simulink library "halout"  (R2021b)
settings: Solver=VariableStepAuto  StartTime=0.0  StopTime=10.0  RelTol=1e-3
undefined symbols (not defined in the file): C_TASK_5MS_S, FALSE, KHAL_CAN1FD1APS3E2E_flg, KHAL_CAN1FD1APS3TxReq_flg, KHAL_CAN1FD1VCU2E2E_flg, KHAL_CAN1FD1VCU2TxReq_flg, KHAL_CAN1FD1VCU3E2E_flg, KHAL_CAN1FD1VCU3TxReq_flg, KHAL_CAN1TxReq_flg, KHAL_CAN1VMCFCM1E2E_flg, KHAL_CAN1VMCFCM1TxReq_flg, KHAL_CAN2TxReq_flg, KHAL_CAN3FD3VCU1toNIDECTxReq_flg, KHAL_CAN3FD3VCU1TxReq_flg, KHAL_CAN3FD3VCU2E2E_flg, KHAL_CAN3FD3VCU2toNIDECE2E_flg, KHAL_CAN3FD3VCU2toNIDECTxReq_flg, KHAL_CAN3FD3VCU2TxReq_flg, KHAL_CAN3TxReq_flg, KHAL_CAN4FD4CE1000E2E_flg, KHAL_CAN4FD4CE1000TxReq_flg, KHAL_CAN4TxReq_flg, KHAL_CAN5TxReq_flg, KHAL_CAN6FD6APS3E2E_flg, KHAL_CAN6FD6APS3TxReq_flg, KHAL_CAN6FD6VCU2E2E_flg, KHAL_CAN6FD6VCU2TxReq_flg, KHAL_CAN6TxReq_flg, ONE_INT, TRUE, ZERO_INT
libraries: FVT_lib x549, simulink x244
(part 4 of 27)

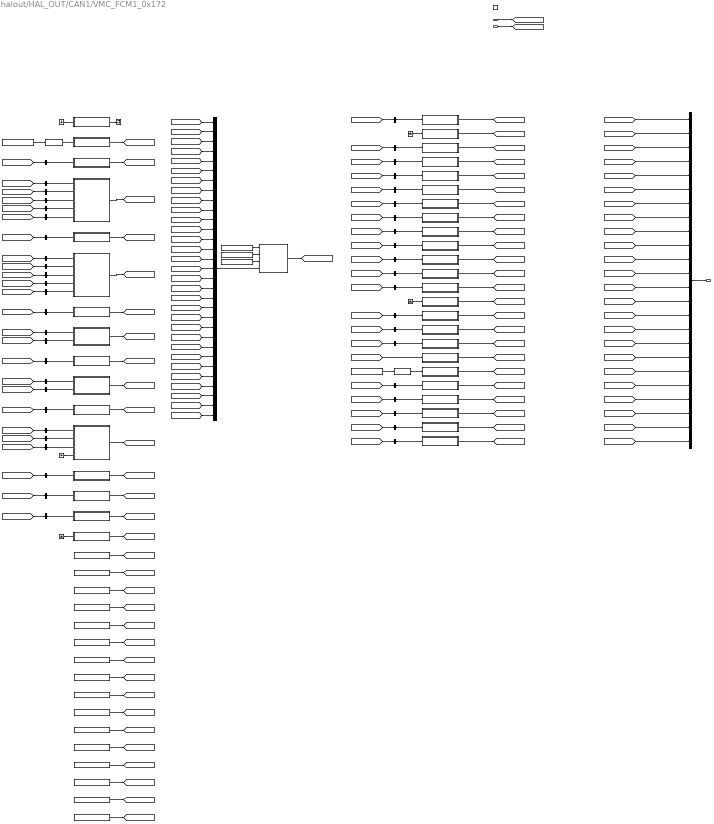
== system halout/HAL_OUT/CAN1/VMC_FCM1_0x172 ==
  BSCP_outputs : Inport  OutDataTypeStr=Bus: BSCP_outputs
  BOUTP_outputs : Inport  Port=2  OutDataTypeStr=Bus: BOUTP_outputs
  Trigger : TriggerPort  TriggerType=function-call  VariantControl=(inherit)
  Byte_0 : Subsystem
  Byte_1 : Subsystem
  Byte_10 : Subsystem
  Byte_11 : Subsystem
  Byte_12 : Subsystem
  Byte_13 : Subsystem
  Byte_14 : Subsystem
  Byte_15 : Subsystem
  Byte_{16..31} (16 alike) : Constant  Value=ZERO_INT
  Byte_2 : Subsystem
  Byte_3 : Subsystem
  Byte_4 : Subsystem
  Byte_5 : Subsystem
  Byte_6 : Subsystem
  Byte_7 : Subsystem
  Byte_8 : Subsystem
  Byte_9 : Subsystem
  CRC8_IfAction_Tx : Subsystem  AncestorBlock=FVT_lib/hal/CRC8_IfAction_Tx
      mask help: MeasumentTrigerEvent
      mask Display: fprintf('CRC8_IfAction');
  Constant : Constant  Value=KHAL_CAN1VMCFCM1E2E_flg
  Constant1 : Constant  Value=0x32
  Constant2 : Constant  Value=0xC9
  Constant3 : Constant  Value=KHAL_CAN1VMCFCM1E2E_flg
  Constant4 : Constant  Value=KHAL_CAN1VMCFCM1E2E_flg
  FDCVMCAngCtrlTqWtGn : Subsystem
  FDCVMCDMSModeCmd : Subsystem
  FDCVMCDrInpTqBstAct : Subsystem
  FDCVMCDrInpTqBstGn : Subsystem
  FDCVMCMaxAngCtrlOutTqLim : Subsystem
  Ground{,1..4} (5 alike) : Ground
  Mux2 : Mux  Inputs=31
  RollingCounter_IfAction : FVT_lib/hal/RollingCounter_IfAction
  RollingCounter_IfAction1 : FVT_lib/hal/RollingCounter_IfAction
  Terminator : Terminator
  VMCACCComfortBandLower : Subsystem
  VMCACCComfortBandUpper : Subsystem
  VMCACCJerkLowerLInit : Subsystem
  VMCACCJerkUpperLInit : Subsystem
  VMCACCRequiredAccel : Subsystem
  VMCACCVehHoldReq : Subsystem
  VMCADASACCSta : Subsystem
  VMCADASAEBReq : Subsystem
  VMCADASAEBSta : Subsystem
  VMCADASDBSReq : Subsystem
  VMCADASFaultSta : Subsystem
  VMCAEBVehHoldReq : Subsystem
  VMCFCM1Checksum : Subsystem
  VMCFCM1LifeCount : Subsystem
  VMCFCMLDWFault : Subsystem
  VMCFCMLDWRequest : Subsystem
  VMCFCMLKAStrToqReq : Subsystem
  VMCFCMLKATOIAct : Subsystem
  VMCFCMLKATOIFault : Subsystem
  bus_creator : BusCreator  Inputs=24  OutDataTypeStr=Bus: DT_CAN1_SG_VMC_FCM1  NonVirtualBus=on
  bus_selector : BusSelector  OutputSignals=VOUTP_LKATOIAct_enum
  bus_selector1 : BusSelector  OutputSignals=VOUTP_AEBVehHoldReq_flg
  bus_selector10 : BusSelector  OutputSignals=VOUTP_ADASDBSReq_enum
  bus_selector11 : BusSelector  OutputSignals=VOUTP_ADASFaultSta_flg
  bus_selector12 : BusSelector  OutputSignals=VOUTP_ACCRequiredAccel_mps2
  bus_selector13 : BusSelector  OutputSignals=VOUTP_ACCComfortBandUpper_mps2
  bus_selector14 : BusSelector  OutputSignals=VOUTP_ACCJerkUpperLimit_mps3
  bus_selector15 : BusSelector  OutputSignals=VOUTP_ACCComfortBandUpper_mps2
  bus_selector16 : BusSelector  OutputSignals=VOUTP_ACCComfortBandLower_mps2
  bus_selector17 : BusSelector  OutputSignals=VOUTP_ACCJerkLowerLimit_mps3
  bus_selector18 : BusSelector  OutputSignals=VOUTP_ACCComfortBandLower_mps2
  bus_selector19 : BusSelector  OutputSignals=VOUTP_FDCVMCDrInpTqBstAct_flg
  bus_selector2 : BusSelector  OutputSignals=VOUTP_FCMLDWFault_flg
  bus_selector20 : BusSelector  OutputSignals=VOUTP_FDCVMCMaxAngCtrlOutTqLim_Nm
  bus_selector21 : BusSelector  OutputSignals=VOUTP_ADASACCSta_enum
  bus_selector22 : BusSelector  OutputSignals=VOUTP_FDCVMCMaxAngCtrlOutTqLim_Nm
  bus_selector23 : BusSelector  OutputSignals=VOUTP_FDCVMCAngCtrlTqWtGn_pct
  bus_selector24 : BusSelector  OutputSignals=VOUTP_FDCVMCDrInpTqBstGn_pct
  bus_selector25 : BusSelector  OutputSignals=VOUTP_FDCVMCAngCtrlTqWtGn_pct
  bus_selector26 : BusSelector  OutputSignals=VOUTP_FDCVMCDrInpTqBstAct_flg
  bus_selector27 : BusSelector  OutputSignals=VOUTP_FDCVMCDrInpTqBstGn_pct
  bus_selector28 : BusSelector  OutputSignals=VOUTP_FDCVMCMaxAngCtrlOutTqLim_Nm
  bus_selector29 : BusSelector  OutputSignals=VOUTP_ACCComfortBandLower_mps2
  bus_selector3 : BusSelector  OutputSignals=VOUTP_FCMLDWRequest_enum
  bus_selector30 : BusSelector  OutputSignals=VOUTP_ACCComfortBandUpper_mps2
  bus_selector31 : BusSelector  OutputSignals=VOUTP_ACCJerkLowerLimit_mps3
  bus_selector32 : BusSelector  OutputSignals=VOUTP_ACCJerkUpperLimit_mps3
  bus_selector33 : BusSelector  OutputSignals=VOUTP_ACCRequiredAccel_mps2
  bus_selector34 : BusSelector  OutputSignals=VOUTP_ACCVehHoldReq_flg
  bus_selector35 : BusSelector  OutputSignals=VOUTP_ADASACCSta_enum
  bus_selector36 : BusSelector  OutputSignals=VOUTP_ADASAEBReq_enum
  bus_selector37 : BusSelector  OutputSignals=VOUTP_ADASDBSReq_enum
  bus_selector38 : BusSelector  OutputSignals=VOUTP_ADASFaultSta_flg
  bus_selector39 : BusSelector  OutputSignals=VOUTP_AEBVehHoldReq_flg
  bus_selector4 : BusSelector  OutputSignals=VOUTP_LKAStrToqReq_Nm
  bus_selector40 : BusSelector  OutputSignals=VOUTP_FCMLDWFault_flg
  bus_selector41 : BusSelector  OutputSignals=VOUTP_FCMLDWRequest_enum
  bus_selector42 : BusSelector  OutputSignals=VOUTP_LKAStrToqReq_Nm
  bus_selector43 : BusSelector  OutputSignals=VOUTP_LKATOIAct_enum
  bus_selector44 : BusSelector  OutputSignals=VOUTP_LKATOIFault_flg
  bus_selector5 : BusSelector  OutputSignals=VOUTP_LKATOIFault_flg
  bus_selector6 : BusSelector  OutputSignals=VOUTP_LKAStrToqReq_Nm
  bus_selector7 : BusSelector  OutputSignals=VOUTP_ACCRequiredAccel_mps2
  bus_selector8 : BusSelector  OutputSignals=VOUTP_ACCVehHoldReq_flg
  bus_selector9 : BusSelector  OutputSignals=VOUTP_ADASAEBReq_enum
  VMC_FCM1 : Outport
  wires:
  BSCP_outputs/1 -> [BSCP_outputs]
  BOUTP_outputs/1 -> [BOUTP_outputs]
  [CAN1_FDC_VMC_AngCtrlTqWtGn] -> bus_creator/1  "CAN1_FDC_VMC_AngCtrlTqWtGn"
  [CAN1_FDC_VMC_DMSMode_Cmd] -> bus_creator/2  "CAN1_FDC_VMC_DMSMode_Cmd"
  [CAN1_FDC_VMC_DrInpTqBstAct] -> bus_creator/3  "CAN1_FDC_VMC_DrInpTqBstAct"
  [CAN1_FDC_VMC_DrInpTqBstGn] -> bus_creator/4  "CAN1_FDC_VMC_DrInpTqBstGn"
  [CAN1_FDC_VMC_MaxAngCtrlOutTqLim] -> bus_creator/5  "CAN1_FDC_VMC_MaxAngCtrlOutTqLim"
  [CAN1_VMC_ACC_ComfortBandLower] -> bus_creator/6  "CAN1_VMC_ACC_ComfortBandLower"
  [CAN1_VMC_ACC_ComfortBandUpper] -> bus_creator/7  "CAN1_VMC_ACC_ComfortBandUpper"
  [CAN1_VMC_ACC_JerkLowerLInit] -> bus_creator/8  "CAN1_VMC_ACC_JerkLowerLInit"
  [CAN1_VMC_ACC_JerkUpperLInit] -> bus_creator/9  "CAN1_VMC_ACC_JerkUpperLInit"
  [CAN1_VMC_ACC_RequiredAccel] -> bus_creator/10  "CAN1_VMC_ACC_RequiredAccel"
  [CAN1_VMC_ACC_VehHoldReq] -> bus_creator/11  "CAN1_VMC_ACC_VehHoldReq"
  [CAN1_VMC_ADAS_ACC_Sta] -> bus_creator/12  "CAN1_VMC_ADAS_ACC_Sta"
  [CAN1_VMC_ADAS_AEBReq] -> bus_creator/13  "CAN1_VMC_ADAS_AEBReq"
  [CAN1_VMC_ADAS_AEB_Sta] -> bus_creator/14  "CAN1_VMC_ADAS_AEB_Sta"
  [CAN1_VMC_ADAS_DBSReq] -> bus_creator/15  "CAN1_VMC_ADAS_DBSReq"
  [CAN1_VMC_ADAS_FaultSta] -> bus_creator/16  "CAN1_VMC_ADAS_FaultSta"
  [CAN1_VMC_AEB_VehHoldReq] -> bus_creator/17  "CAN1_VMC_AEB_VehHoldReq"
  [CAN1_VMC_FCM1_Checksum] -> bus_creator/18  "CAN1_VMC_FCM1_Checksum"
  [CAN1_VMC_FCM1_LifeCount] -> bus_creator/19  "CAN1_VMC_FCM1_LifeCount"
  [CAN1_VMC_FCM_LDW_Fault] -> bus_creator/20  "CAN1_VMC_FCM_LDW_Fault"
  [CAN1_VMC_FCM_LDW_Request] -> bus_creator/21  "CAN1_VMC_FCM_LDW_Request"
  [CAN1_VMC_FCM_LKA_StrToqReq] -> bus_creator/22  "CAN1_VMC_FCM_LKA_StrToqReq"
  [CAN1_VMC_FCM_LKA_TOIAct] -> bus_creator/23  "CAN1_VMC_FCM_LKA_TOIAct"
  [CAN1_VMC_FCM_LKA_TOIFault] -> bus_creator/24  "CAN1_VMC_FCM_LKA_TOIFault"
  bus_creator/1 -> VMC_FCM1/1
  FDCVMCAngCtrlTqWtGn/1(CAN1_FDC_VMC_AngCtrlTqWtGn) -> [CAN1_FDC_VMC_AngCtrlTqWtGn]
  FDCVMCDMSModeCmd/1(CAN1_FDC_VMC_DMSMode_Cmd) -> [CAN1_FDC_VMC_DMSMode_Cmd]
  FDCVMCDrInpTqBstAct/1(CAN1_FDC_VMC_DrInpTqBstAct) -> [CAN1_FDC_VMC_DrInpTqBstAct]
  FDCVMCDrInpTqBstGn/1(CAN1_FDC_VMC_DrInpTqBstGn) -> [CAN1_FDC_VMC_DrInpTqBstGn]
  FDCVMCMaxAngCtrlOutTqLim/1(CAN1_FDC_VMC_MaxAngCtrlOutTqLim) -> [CAN1_FDC_VMC_MaxAngCtrlOutTqLim]
  VMCACCComfortBandLower/1(CAN1_VMC_ACC_ComfortBandLower) -> [CAN1_VMC_ACC_ComfortBandLower]
  VMCACCComfortBandUpper/1(CAN1_VMC_ACC_ComfortBandUpper) -> [CAN1_VMC_ACC_ComfortBandUpper]
  VMCACCJerkLowerLInit/1(CAN1_VMC_ACC_JerkLowerLInit) -> [CAN1_VMC_ACC_JerkLowerLInit]
  VMCACCJerkUpperLInit/1(CAN1_VMC_ACC_JerkUpperLInit) -> [CAN1_VMC_ACC_JerkUpperLInit]
  VMCACCRequiredAccel/1(CAN1_VMC_ACC_RequiredAccel) -> [CAN1_VMC_ACC_RequiredAccel]
  VMCACCVehHoldReq/1(CAN1_VMC_ACC_VehHoldReq) -> [CAN1_VMC_ACC_VehHoldReq]
  VMCADASACCSta/1(CAN1_VMC_ADAS_ACC_Sta) -> [CAN1_VMC_ADAS_ACC_Sta]
  VMCADASAEBReq/1(CAN1_VMC_ADAS_AEBReq) -> [CAN1_VMC_ADAS_AEBReq]
  VMCADASAEBSta/1(CAN1_VMC_ADAS_AEB_Sta) -> [CAN1_VMC_ADAS_AEB_Sta]
  VMCADASDBSReq/1(CAN1_VMC_ADAS_DBSReq) -> [CAN1_VMC_ADAS_DBSReq]
  VMCADASFaultSta/1(CAN1_VMC_ADAS_FaultSta) -> [CAN1_VMC_ADAS_FaultSta]
  VMCAEBVehHoldReq/1(CAN1_VMC_AEB_VehHoldReq) -> [CAN1_VMC_AEB_VehHoldReq]
  VMCFCM1Checksum/1(CAN1_VMC_FCM1_Checksum) -> [CAN1_VMC_FCM1_Checksum]
  VMCFCM1LifeCount/1(CAN1_VMC_FCM1_LifeCount) -> [CAN1_VMC_FCM1_LifeCount]
  VMCFCMLDWFault/1(CAN1_VMC_FCM_LDW_Fault) -> [CAN1_VMC_FCM_LDW_Fault]
  VMCFCMLDWRequest/1(CAN1_VMC_FCM_LDW_Request) -> [CAN1_VMC_FCM_LDW_Request]
  VMCFCMLKAStrToqReq/1(CAN1_VMC_FCM_LKA_StrToqReq) -> [CAN1_VMC_FCM_LKA_StrToqReq]
  VMCFCMLKATOIAct/1(CAN1_VMC_FCM_LKA_TOIAct) -> [CAN1_VMC_FCM_LKA_TOIAct]
  VMCFCMLKATOIFault/1(CAN1_VMC_FCM_LKA_TOIFault) -> [CAN1_VMC_FCM_LKA_TOIFault]
  Byte_0/1(Byte_0) -> Terminator/1
  Byte_1/1(Byte_1) -> [Byte_1]
  Byte_2/1(Byte_2) -> [Byte_2]
  Byte_3/1(Byte_3) -> [Byte_3]
  Byte_4/1(Byte_4) -> [Byte_4]
  Byte_5/1(Byte_5) -> [Byte_5]
  Byte_6/1(Byte_6) -> [Byte_6]
  Byte_7/1(Byte_7) -> [Byte_7]
  Byte_8/1(Byte_8) -> [Byte_8]
  Byte_9/1(Byte_9) -> [Byte_9]
  Byte_10/1(Byte_10) -> [Byte_10]
  Byte_11/1(Byte_11) -> [Byte_11]
  Byte_12/1(Byte_12) -> [Byte_12]
  Byte_13/1(Byte_13) -> [Byte_13]
  Byte_14/1(Byte_14) -> [Byte_14]
  Byte_15/1(Byte_15) -> [Byte_15]
  Byte_16/1 -> [Byte_16]
  Byte_17/1 -> [Byte_17]
  Byte_18/1 -> [Byte_18]
  Byte_19/1 -> [Byte_19]
  Byte_20/1 -> [Byte_20]
  Byte_21/1 -> [Byte_21]
  Byte_22/1 -> [Byte_22]
  Byte_23/1 -> [Byte_23]
  Byte_24/1 -> [Byte_24]
  Byte_25/1 -> [Byte_25]
  Byte_26/1 -> [Byte_26]
  Byte_27/1 -> [Byte_27]
  Byte_28/1 -> [Byte_28]
  Byte_29/1 -> [Byte_29]
  Byte_30/1 -> [Byte_30]
  Byte_31/1 -> [Byte_31]
  Mux2/1 -> CRC8_IfAction_Tx/4(RawData)
  Constant/1 -> CRC8_IfAction_Tx/1(CAN_E2E_flg)
  Constant1/1 -> CRC8_IfAction_Tx/2(DataID1)
  Constant2/1 -> CRC8_IfAction_Tx/3(DataID2)
  CRC8_IfAction_Tx/1(CRC8) -> [VMC_FCM1_Checksum]
  Ground/1 -> Byte_0/1(VMC_FCM1_Checksum)
  [Byte_1] -> Mux2/1
  RollingCounter_IfAction/1 -> Byte_1/1(VMC_FCM1_LifeCount)
  Constant3/1 -> RollingCounter_IfAction/1
  [Byte_2] -> Mux2/2
  bus_selector/1 -> Byte_2/1(VMC_FCM_LKA_TOIAct)  "<VOUTP_LKATOIAct_enum>"
  [BOUTP_outputs] -> bus_selector/1
  [Byte_3] -> Mux2/3
  bus_selector1/1 -> Byte_3/1(VMC_AEB_VehHoldReq)  "<VOUTP_AEBVehHoldReq_flg>"
  [BOUTP_outputs] -> bus_selector1/1
  bus_selector2/1 -> Byte_3/2(VMC_FCM_LDW_Fault)  "<VOUTP_FCMLDWFault_flg>"
  [BOUTP_outputs] -> bus_selector2/1
  bus_selector3/1 -> Byte_3/3(VMC_FCM_LDW_Request)  "<VOUTP_FCMLDWRequest_enum>"
  [BOUTP_outputs] -> bus_selector3/1
  bus_selector4/1 -> Byte_3/4(VMC_FCM_LKA_StrToqReq)  "<VOUTP_LKAStrToqReq_Nm>"
  [BOUTP_outputs] -> bus_selector4/1
  bus_selector5/1 -> Byte_3/5(VMC_FCM_LKA_TOIFault)  "<VOUTP_LKATOIFault_flg>"
  [BOUTP_outputs] -> bus_selector5/1
  [Byte_4] -> Mux2/4
  bus_selector6/1 -> Byte_4/1(VMC_FCM_LKA_StrToqReq)  "<VOUTP_LKAStrToqReq_Nm>"
  [BOUTP_outputs] -> bus_selector6/1
  [Byte_5] -> Mux2/5
  bus_selector7/1 -> Byte_5/1(VMC_ACC_RequiredAccel)  "<VOUTP_ACCRequiredAccel_mps2>"
  [BOUTP_outputs] -> bus_selector7/1
  bus_selector8/1 -> Byte_5/2(VMC_ACC_VehHoldReq)  "<VOUTP_ACCVehHoldReq_flg>"
  [BOUTP_outputs] -> bus_selector8/1
  bus_selector9/1 -> Byte_5/3(VMC_ADAS_AEBReq)  "<VOUTP_ADASAEBReq_enum>"
  [BOUTP_outputs] -> bus_selector9/1
  bus_selector10/1 -> Byte_5/4(VMC_ADAS_DBSReq)  "<VOUTP_ADASDBSReq_enum>"
  [BOUTP_outputs] -> bus_selector10/1
  bus_selector11/1 -> Byte_5/5(VMC_ADAS_FaultSta)  "<VOUTP_ADASFaultSta_flg>"
  [BOUTP_outputs] -> bus_selector11/1
  [Byte_6] -> Mux2/6
  bus_selector12/1 -> Byte_6/1(VMC_ACC_RequiredAccel)  "<VOUTP_ACCRequiredAccel_mps2>"
  [BOUTP_outputs] -> bus_selector12/1
  [Byte_7] -> Mux2/7
  bus_selector13/1 -> Byte_7/1(VMC_ACC_ComfortBandUpper)  "<VOUTP_ACCComfortBandUpper_mps2>"
  [BOUTP_outputs] -> bus_selector13/1
  bus_selector14/1 -> Byte_7/2(VMC_ACC_JerkUpperLInit)  "<VOUTP_ACCJerkUpperLimit_mps3>"
  [BOUTP_outputs] -> bus_selector14/1
  [Byte_8] -> Mux2/8
  bus_selector15/1 -> Byte_8/1(VMC_ACC_ComfortBandUpper)  "<VOUTP_ACCComfortBandUpper_mps2>"
  [BOUTP_outputs] -> bus_selector15/1
  [Byte_9] -> Mux2/9
  bus_selector16/1 -> Byte_9/1(VMC_ACC_ComfortBandLower)  "<VOUTP_ACCComfortBandLower_mps2>"
  [BOUTP_outputs] -> bus_selector16/1
  bus_selector17/1 -> Byte_9/2(VMC_ACC_JerkLowerLInit)  "<VOUTP_ACCJerkLowerLimit_mps3>"
  [BOUTP_outputs] -> bus_selector17/1
  [Byte_10] -> Mux2/10
  bus_selector18/1 -> Byte_10/1(VMC_ACC_ComfortBandLower)  "<VOUTP_ACCComfortBandLower_mps2>"
  [BOUTP_outputs] -> bus_selector18/1
  [Byte_11] -> Mux2/11
  bus_selector19/1 -> Byte_11/1(FDC_VMC_DrInpTqBstAct)  "<VOUTP_FDCVMCDrInpTqBstAct_flg>"
  [BOUTP_outputs] -> bus_selector19/1
  bus_selector20/1 -> Byte_11/2(FDC_VMC_MaxAngCtrlOutTqLim)  "<VOUTP_FDCVMCMaxAngCtrlOutTqLim_Nm>"
  [BOUTP_outputs] -> bus_selector20/1
  bus_selector21/1 -> Byte_11/3(VMC_ADAS_ACC_Sta)  "<VOUTP_ADASACCSta_enum>"
  [BOUTP_outputs] -> bus_selector21/1
  Ground1/1 -> Byte_11/4(VMC_ADAS_AEB_Sta)
  [Byte_12] -> Mux2/12
  bus_selector22/1 -> Byte_12/1(FDC_VMC_MaxAngCtrlOutTqLim)  "<VOUTP_FDCVMCMaxAngCtrlOutTqLim_Nm>"
  [BOUTP_outputs] -> bus_selector22/1
  [Byte_13] -> Mux2/13
  bus_selector23/1 -> Byte_13/1(FDC_VMC_AngCtrlTqWtGn)  "<VOUTP_FDCVMCAngCtrlTqWtGn_pct>"
  [BOUTP_outputs] -> bus_selector23/1
  [Byte_14] -> Mux2/14
  bus_selector24/1 -> Byte_14/1(FDC_VMC_DrInpTqBstGn)  "<VOUTP_FDCVMCDrInpTqBstGn_pct>"
  [BOUTP_outputs] -> bus_selector24/1
  [Byte_15] -> Mux2/15
  Ground2/1 -> Byte_15/1(FDC_VMC_DMSMode_Cmd)
  [Byte_16] -> Mux2/16
  [Byte_17] -> Mux2/17
  [Byte_18] -> Mux2/18
  [Byte_19] -> Mux2/19
  [Byte_20] -> Mux2/20
  [Byte_21] -> Mux2/21
  [Byte_22] -> Mux2/22
  [Byte_23] -> Mux2/23
  [Byte_24] -> Mux2/24
  [Byte_25] -> Mux2/25
  [Byte_26] -> Mux2/26
  [Byte_27] -> Mux2/27
  [Byte_28] -> Mux2/28
  [Byte_29] -> Mux2/29
  [Byte_30] -> Mux2/30
  [Byte_31] -> Mux2/31
  bus_selector25/1 -> FDCVMCAngCtrlTqWtGn/1(FDCVMCAngCtrlTqWtGn)  "<VOUTP_FDCVMCAngCtrlTqWtGn_pct>"
  [BOUTP_outputs] -> bus_selector25/1
  Ground3/1 -> FDCVMCDMSModeCmd/1(FDCVMCDMSModeCmd)
  bus_selector26/1 -> FDCVMCDrInpTqBstAct/1(FDCVMCDrInpTqBstAct)  "<VOUTP_FDCVMCDrInpTqBstAct_flg>"
  [BOUTP_outputs] -> bus_selector26/1
  bus_selector27/1 -> FDCVMCDrInpTqBstGn/1(FDCVMCDrInpTqBstGn)  "<VOUTP_FDCVMCDrInpTqBstGn_pct>"
  [BOUTP_outputs] -> bus_selector27/1
  bus_selector28/1 -> FDCVMCMaxAngCtrlOutTqLim/1(FDCVMCMaxAngCtrlOutTqLim)  "<VOUTP_FDCVMCMaxAngCtrlOutTqLim_Nm>"
  [BOUTP_outputs] -> bus_selector28/1
  bus_selector29/1 -> VMCACCComfortBandLower/1(VMCACCComfortBandLower)  "<VOUTP_ACCComfortBandLower_mps2>"
  [BOUTP_outputs] -> bus_selector29/1
  bus_selector30/1 -> VMCACCComfortBandUpper/1(VMCACCComfortBandUpper)  "<VOUTP_ACCComfortBandUpper_mps2>"
  [BOUTP_outputs] -> bus_selector30/1
  bus_selector31/1 -> VMCACCJerkLowerLInit/1(VMCACCJerkLowerLInit)  "<VOUTP_ACCJerkLowerLimit_mps3>"
  [BOUTP_outputs] -> bus_selector31/1
  bus_selector32/1 -> VMCACCJerkUpperLInit/1(VMCACCJerkUpperLInit)  "<VOUTP_ACCJerkUpperLimit_mps3>"
  [BOUTP_outputs] -> bus_selector32/1
  bus_selector33/1 -> VMCACCRequiredAccel/1(VMCACCRequiredAccel)  "<VOUTP_ACCRequiredAccel_mps2>"
  [BOUTP_outputs] -> bus_selector33/1
  bus_selector34/1 -> VMCACCVehHoldReq/1(VMCACCVehHoldReq)  "<VOUTP_ACCVehHoldReq_flg>"
  [BOUTP_outputs] -> bus_selector34/1
  bus_selector35/1 -> VMCADASACCSta/1(VMCADASACCSta)  "<VOUTP_ADASACCSta_enum>"
  [BOUTP_outputs] -> bus_selector35/1
  bus_selector36/1 -> VMCADASAEBReq/1(VMCADASAEBReq)  "<VOUTP_ADASAEBReq_enum>"
  [BOUTP_outputs] -> bus_selector36/1
  Ground4/1 -> VMCADASAEBSta/1(VMCADASAEBSta)
  bus_selector37/1 -> VMCADASDBSReq/1(VMCADASDBSReq)  "<VOUTP_ADASDBSReq_enum>"
  [BOUTP_outputs] -> bus_selector37/1
  bus_selector38/1 -> VMCADASFaultSta/1(VMCADASFaultSta)  "<VOUTP_ADASFaultSta_flg>"
  [BOUTP_outputs] -> bus_selector38/1
  bus_selector39/1 -> VMCAEBVehHoldReq/1(VMCAEBVehHoldReq)  "<VOUTP_AEBVehHoldReq_flg>"
  [BOUTP_outputs] -> bus_selector39/1
  [VMC_FCM1_Checksum] -> VMCFCM1Checksum/1(VMCFCM1Checksum)
  RollingCounter_IfAction1/1 -> VMCFCM1LifeCount/1(VMCFCM1LifeCount)
  Constant4/1 -> RollingCounter_IfAction1/1
  bus_selector40/1 -> VMCFCMLDWFault/1(VMCFCMLDWFault)  "<VOUTP_FCMLDWFault_flg>"
  [BOUTP_outputs] -> bus_selector40/1
  bus_selector41/1 -> VMCFCMLDWRequest/1(VMCFCMLDWRequest)  "<VOUTP_FCMLDWRequest_enum>"
  [BOUTP_outputs] -> bus_selector41/1
  bus_selector42/1 -> VMCFCMLKAStrToqReq/1(VMCFCMLKAStrToqReq)  "<VOUTP_LKAStrToqReq_Nm>"
  [BOUTP_outputs] -> bus_selector42/1
  bus_selector43/1 -> VMCFCMLKATOIAct/1(VMCFCMLKATOIAct)  "<VOUTP_LKATOIAct_enum>"
  [BOUTP_outputs] -> bus_selector43/1
  bus_selector44/1 -> VMCFCMLKATOIFault/1(VMCFCMLKATOIFault)  "<VOUTP_LKATOIFault_flg>"
  [BOUTP_outputs] -> bus_selector44/1

== system halout/HAL_OUT/CAN1/VMC_FCM1_Tx ==
  TxReq : Inport
  Chart : Stateflow chart  TreatAsAtomicUnit=on
  Constant : Constant  Value=C_TASK_5MS_S
  Constant3 : Constant  Value=CycleTime
  Data Type Conversion : DataTypeConversion  OutDataTypeStr=uint16
  Divide : Product  Inputs=*/
  Gain : Gain  Gain=0.001
  TxTrigger : Outport
  wires:
  Data Type Conversion/1 -> Chart/2(CycleCnt)
  Constant3/1 -> Gain/1
  Gain/1 -> Divide/1
  Chart/1(TxTrigger()) -> TxTrigger/1
  Divide/1 -> Data Type Conversion/1
  TxReq/1 -> Chart/1(TxReq)
  Constant/1 -> Divide/2

== system halout/HAL_OUT/CAN2/FD2_C20_0_0x210 ==
  BSCP_outputs : Inport  OutDataTypeStr=Bus: BSCP_outputs
  BOUTP_outputs : Inport  Port=2  OutDataTypeStr=Bus: BOUTP_outputs
  APSExitCondition : Subsystem
  APSRQDisplay : Subsystem
  APSSWVer : Subsystem
  APSStaSystem : Subsystem
  CAASSta : Subsystem
  DISCDISCTargetSpd : Subsystem
  FDCVCURegenLimIndSta : Subsystem
  FDCVCURegenModeSta : Subsystem
  FDCVCUSmartEcoSpdLimSta : Subsystem
  FDCVCUSmartEcoSta : Subsystem
  FDCVMCSetSpdDispSta : Subsystem
  FDCVMCSetSpdSta : Subsystem
  FDCVMCSpdCtrlModeSta : Subsystem
  FDCVMCSpdCtrlSta : Subsystem
  Ground : Ground
  Ground1 : Ground
  PASAFCL : Subsystem
  PASAFCR : Subsystem
  PASAFML : Subsystem
  PASAFMR : Subsystem
  PASARCL : Subsystem
  PASARCR : Subsystem
  PASARML : Subsystem
  PASARMR : Subsystem
  PASChime : Subsystem
  PASDFCL : Subsystem
  PASDFCR : Subsystem
  PASDFML : Subsystem
  PASDFMR : Subsystem
  PASDRCL : Subsystem
  PASDRCR : Subsystem
  PASDRML : Subsystem
  PASDRMR : Subsystem
  PASSNSRLayout : Subsystem
  USSStaFCL : Subsystem
  USSStaFCR : Subsystem
  USSStaFLL : Subsystem
  USSStaFLR : Subsystem
  USSStaFML : Subsystem
  USSStaFMR : Subsystem
  USSStaRCL : Subsystem
  USSStaRCR : Subsystem
  USSStaRLL : Subsystem
  USSStaRLR : Subsystem
  USSStaRML : Subsystem
  USSStaRMR : Subsystem
  VMCVCUCCCrlSta : Subsystem
  VMCVCUMSACrlSta : Subsystem
  bus_creator : BusCreator  Inputs=46  OutDataTypeStr=Bus: DT_CAN2_SG_FD2_C20_0  NonVirtualBus=on
  bus_selector : BusSelector  OutputSignals=VOUTP_APSExitCondition_enum
  bus_selector1 : BusSelector  OutputSignals=VOUTP_APSRQDisplay_enum
  bus_selector10 : BusSelector  OutputSignals=VOUTP_SpdCtrlMode_enum
  bus_selector11 : BusSelector  OutputSignals=VOUTP_SpdCtrlSta_flg
  bus_selector12 : BusSelector  OutputSignals=VOUTP_PASAFCL_enum
  bus_selector13 : BusSelector  OutputSignals=VOUTP_PASAFCR_enum
  bus_selector14 : BusSelector  OutputSignals=VOUTP_PASAFML_enum
  bus_selector15 : BusSelector  OutputSignals=VOUTP_PASAFMR_enum
  bus_selector16 : BusSelector  OutputSignals=VOUTP_PASARCL_enum
  bus_selector17 : BusSelector  OutputSignals=VOUTP_PASARCR_enum
  bus_selector18 : BusSelector  OutputSignals=VOUTP_PASARML_enum
  bus_selector19 : BusSelector  OutputSignals=VOUTP_PASARMR_enum
  bus_selector2 : BusSelector  OutputSignals=VOUTP_APSSWVer_enum
  bus_selector20 : BusSelector  OutputSignals=VOUTP_Chime_enum
  bus_selector21 : BusSelector  OutputSignals=VOUTP_PASDFCL_cm
  bus_selector22 : BusSelector  OutputSignals=VOUTP_PASDFCR_cm
  bus_selector23 : BusSelector  OutputSignals=VOUTP_PASDFML_cm
  bus_selector24 : BusSelector  OutputSignals=VOUTP_PASDFMR_cm
  bus_selector25 : BusSelector  OutputSignals=VOUTP_PASDRCL_cm
  bus_selector26 : BusSelector  OutputSignals=VOUTP_PASDRCR_cm
  bus_selector27 : BusSelector  OutputSignals=VOUTP_PASDRML_cm
  bus_selector28 : BusSelector  OutputSignals=VOUTP_PASDRMR_cm
  bus_selector29 : BusSelector  OutputSignals=VOUTP_SNSRLayout_enum
  bus_selector3 : BusSelector  OutputSignals=VOUTP_APSStaSys_enum
  bus_selector30 : BusSelector  OutputSignals=VOUTP_USSStaFCL_flg
  bus_selector31 : BusSelector  OutputSignals=VOUTP_USSStaFCR_flg
  bus_selector32 : BusSelector  OutputSignals=VOUTP_USSStaFLL_flg
  bus_selector33 : BusSelector  OutputSignals=VOUTP_USSStaFLR_flg
  bus_selector34 : BusSelector  OutputSignals=VOUTP_USSStaFML_flg
  bus_selector35 : BusSelector  OutputSignals=VOUTP_USSStaFMR_flg
  bus_selector36 : BusSelector  OutputSignals=VOUTP_USSStaRCL_flg
  bus_selector37 : BusSelector  OutputSignals=VOUTP_USSStaRCR_flg
  bus_selector38 : BusSelector  OutputSignals=VOUTP_USSStaRLL_flg
  bus_selector39 : BusSelector  OutputSignals=VOUTP_USSStaRLR_flg
  bus_selector4 : BusSelector  OutputSignals=VOUTP_CAASSta_enum
  bus_selector40 : BusSelector  OutputSignals=VOUTP_USSStaRML_flg
  bus_selector41 : BusSelector  OutputSignals=VOUTP_USSStaRMR_flg
  bus_selector42 : BusSelector  OutputSignals=VOUTP_CCCtrlSta_enum
  bus_selector43 : BusSelector  OutputSignals=VOUTP_MSACtrlSta_enum
  bus_selector5 : BusSelector  OutputSignals=VOUTP_DISCTargetSpd_kph
  bus_selector6 : BusSelector  OutputSignals=VOUTP_RegenLimIndSta_flg
  bus_selector7 : BusSelector  OutputSignals=VOUTP_FDCVCURegenMode_enum
  bus_selector8 : BusSelector  OutputSignals=VOUTP_SetSpdLimWarn_flg
  bus_selector9 : BusSelector  OutputSignals=VOUTP_SetSpd_kph
  FD2_C20_0 : Outport
  wires:
  BSCP_outputs/1 -> [BSCP_outputs]
  BOUTP_outputs/1 -> [BOUTP_outputs]
  [CAN2_APS_ExitCondition] -> bus_creator/1  "CAN2_APS_ExitCondition"
  [CAN2_APS_RQ_Display] -> bus_creator/2  "CAN2_APS_RQ_Display"
  [CAN2_APS_SW_Ver] -> bus_creator/3  "CAN2_APS_SW_Ver"
  [CAN2_APS_Sta_System] -> bus_creator/4  "CAN2_APS_Sta_System"
  [CAN2_CAAS_Sta] -> bus_creator/5  "CAN2_CAAS_Sta"
  [CAN2_DISC_DISCTargetSpd] -> bus_creator/6  "CAN2_DISC_DISCTargetSpd"
  [CAN2_FDC_VCU_RegenLimInd_Sta] -> bus_creator/7  "CAN2_FDC_VCU_RegenLimInd_Sta"
  [CAN2_FDC_VCU_RegenMode_Sta] -> bus_creator/8  "CAN2_FDC_VCU_RegenMode_Sta"
  [CAN2_FDC_VCU_SmartEcoSpdLim_Sta] -> bus_creator/9  "CAN2_FDC_VCU_SmartEcoSpdLim_Sta"
  [CAN2_FDC_VCU_SmartEco_Sta] -> bus_creator/10  "CAN2_FDC_VCU_SmartEco_Sta"
  [CAN2_FDC_VMC_SetSpdDisp_Sta] -> bus_creator/11  "CAN2_FDC_VMC_SetSpdDisp_Sta"
  [CAN2_FDC_VMC_SetSpd_Sta] -> bus_creator/12  "CAN2_FDC_VMC_SetSpd_Sta"
  [CAN2_FDC_VMC_SpdCtrlMode_Sta] -> bus_creator/13  "CAN2_FDC_VMC_SpdCtrlMode_Sta"
  [CAN2_FDC_VMC_SpdCtrl_Sta] -> bus_creator/14  "CAN2_FDC_VMC_SpdCtrl_Sta"
  [CAN2_PAS_A_FCL] -> bus_creator/15  "CAN2_PAS_A_FCL"
  [CAN2_PAS_A_FCR] -> bus_creator/16  "CAN2_PAS_A_FCR"
  [CAN2_PAS_A_FML] -> bus_creator/17  "CAN2_PAS_A_FML"
  [CAN2_PAS_A_FMR] -> bus_creator/18  "CAN2_PAS_A_FMR"
  [CAN2_PAS_A_RCL] -> bus_creator/19  "CAN2_PAS_A_RCL"
  [CAN2_PAS_A_RCR] -> bus_creator/20  "CAN2_PAS_A_RCR"
  [CAN2_PAS_A_RML] -> bus_creator/21  "CAN2_PAS_A_RML"
  [CAN2_PAS_A_RMR] -> bus_creator/22  "CAN2_PAS_A_RMR"
  [CAN2_PAS_Chime] -> bus_creator/23  "CAN2_PAS_Chime"
  [CAN2_PAS_D_FCL] -> bus_creator/24  "CAN2_PAS_D_FCL"
  [CAN2_PAS_D_FCR] -> bus_creator/25  "CAN2_PAS_D_FCR"
  [CAN2_PAS_D_FML] -> bus_creator/26  "CAN2_PAS_D_FML"
  [CAN2_PAS_D_FMR] -> bus_creator/27  "CAN2_PAS_D_FMR"
  [CAN2_PAS_D_RCL] -> bus_creator/28  "CAN2_PAS_D_RCL"
  [CAN2_PAS_D_RCR] -> bus_creator/29  "CAN2_PAS_D_RCR"
  [CAN2_PAS_D_RML] -> bus_creator/30  "CAN2_PAS_D_RML"
  [CAN2_PAS_D_RMR] -> bus_creator/31  "CAN2_PAS_D_RMR"
  [CAN2_PAS_SNSR_Layout] -> bus_creator/32  "CAN2_PAS_SNSR_Layout"
  [CAN2_USS_Sta_FCL] -> bus_creator/33  "CAN2_USS_Sta_FCL"
  [CAN2_USS_Sta_FCR] -> bus_creator/34  "CAN2_USS_Sta_FCR"
  [CAN2_USS_Sta_FLL] -> bus_creator/35  "CAN2_USS_Sta_FLL"
  [CAN2_USS_Sta_FLR] -> bus_creator/36  "CAN2_USS_Sta_FLR"
  [CAN2_USS_Sta_FML] -> bus_creator/37  "CAN2_USS_Sta_FML"
  [CAN2_USS_Sta_FMR] -> bus_creator/38  "CAN2_USS_Sta_FMR"
  [CAN2_USS_Sta_RCL] -> bus_creator/39  "CAN2_USS_Sta_RCL"
  [CAN2_USS_Sta_RCR] -> bus_creator/40  "CAN2_USS_Sta_RCR"
  [CAN2_USS_Sta_RLL] -> bus_creator/41  "CAN2_USS_Sta_RLL"
  [CAN2_USS_Sta_RLR] -> bus_creator/42  "CAN2_USS_Sta_RLR"
  [CAN2_USS_Sta_RML] -> bus_creator/43  "CAN2_USS_Sta_RML"
  [CAN2_USS_Sta_RMR] -> bus_creator/44  "CAN2_USS_Sta_RMR"
  [CAN2_VMC_VCU_CC_Crl_Sta] -> bus_creator/45  "CAN2_VMC_VCU_CC_Crl_Sta"
  [CAN2_VMC_VCU_MSA_Crl_Sta] -> bus_creator/46  "CAN2_VMC_VCU_MSA_Crl_Sta"
  bus_creator/1 -> FD2_C20_0/1
  APSExitCondition/1(CAN2_APS_ExitCondition) -> [CAN2_APS_ExitCondition]
  APSRQDisplay/1(CAN2_APS_RQ_Display) -> [CAN2_APS_RQ_Display]
  APSSWVer/1(CAN2_APS_SW_Ver) -> [CAN2_APS_SW_Ver]
  APSStaSystem/1(CAN2_APS_Sta_System) -> [CAN2_APS_Sta_System]
  CAASSta/1(CAN2_CAAS_Sta) -> [CAN2_CAAS_Sta]
  DISCDISCTargetSpd/1(CAN2_DISC_DISCTargetSpd) -> [CAN2_DISC_DISCTargetSpd]
  FDCVCURegenLimIndSta/1(CAN2_FDC_VCU_RegenLimInd_Sta) -> [CAN2_FDC_VCU_RegenLimInd_Sta]
  FDCVCURegenModeSta/1(CAN2_FDC_VCU_RegenMode_Sta) -> [CAN2_FDC_VCU_RegenMode_Sta]
  FDCVCUSmartEcoSpdLimSta/1(CAN2_FDC_VCU_SmartEcoSpdLim_Sta) -> [CAN2_FDC_VCU_SmartEcoSpdLim_Sta]
  FDCVCUSmartEcoSta/1(CAN2_FDC_VCU_SmartEco_Sta) -> [CAN2_FDC_VCU_SmartEco_Sta]
  FDCVMCSetSpdDispSta/1(CAN2_FDC_VMC_SetSpdDisp_Sta) -> [CAN2_FDC_VMC_SetSpdDisp_Sta]
  FDCVMCSetSpdSta/1(CAN2_FDC_VMC_SetSpd_Sta) -> [CAN2_FDC_VMC_SetSpd_Sta]
  FDCVMCSpdCtrlModeSta/1(CAN2_FDC_VMC_SpdCtrlMode_Sta) -> [CAN2_FDC_VMC_SpdCtrlMode_Sta]
  FDCVMCSpdCtrlSta/1(CAN2_FDC_VMC_SpdCtrl_Sta) -> [CAN2_FDC_VMC_SpdCtrl_Sta]
  PASAFCL/1(CAN2_PAS_A_FCL) -> [CAN2_PAS_A_FCL]
  PASAFCR/1(CAN2_PAS_A_FCR) -> [CAN2_PAS_A_FCR]
  PASAFML/1(CAN2_PAS_A_FML) -> [CAN2_PAS_A_FML]
  PASAFMR/1(CAN2_PAS_A_FMR) -> [CAN2_PAS_A_FMR]
  PASARCL/1(CAN2_PAS_A_RCL) -> [CAN2_PAS_A_RCL]
  PASARCR/1(CAN2_PAS_A_RCR) -> [CAN2_PAS_A_RCR]
  PASARML/1(CAN2_PAS_A_RML) -> [CAN2_PAS_A_RML]
  PASARMR/1(CAN2_PAS_A_RMR) -> [CAN2_PAS_A_RMR]
  PASChime/1(CAN2_PAS_Chime) -> [CAN2_PAS_Chime]
  PASDFCL/1(CAN2_PAS_D_FCL) -> [CAN2_PAS_D_FCL]
  PASDFCR/1(CAN2_PAS_D_FCR) -> [CAN2_PAS_D_FCR]
  PASDFML/1(CAN2_PAS_D_FML) -> [CAN2_PAS_D_FML]
  PASDFMR/1(CAN2_PAS_D_FMR) -> [CAN2_PAS_D_FMR]
  PASDRCL/1(CAN2_PAS_D_RCL) -> [CAN2_PAS_D_RCL]
  PASDRCR/1(CAN2_PAS_D_RCR) -> [CAN2_PAS_D_RCR]
  PASDRML/1(CAN2_PAS_D_RML) -> [CAN2_PAS_D_RML]
  PASDRMR/1(CAN2_PAS_D_RMR) -> [CAN2_PAS_D_RMR]
  PASSNSRLayout/1(CAN2_PAS_SNSR_Layout) -> [CAN2_PAS_SNSR_Layout]
  USSStaFCL/1(CAN2_USS_Sta_FCL) -> [CAN2_USS_Sta_FCL]
  USSStaFCR/1(CAN2_USS_Sta_FCR) -> [CAN2_USS_Sta_FCR]
  USSStaFLL/1(CAN2_USS_Sta_FLL) -> [CAN2_USS_Sta_FLL]
  USSStaFLR/1(CAN2_USS_Sta_FLR) -> [CAN2_USS_Sta_FLR]
  USSStaFML/1(CAN2_USS_Sta_FML) -> [CAN2_USS_Sta_FML]
  USSStaFMR/1(CAN2_USS_Sta_FMR) -> [CAN2_USS_Sta_FMR]
  USSStaRCL/1(CAN2_USS_Sta_RCL) -> [CAN2_USS_Sta_RCL]
  USSStaRCR/1(CAN2_USS_Sta_RCR) -> [CAN2_USS_Sta_RCR]
  USSStaRLL/1(CAN2_USS_Sta_RLL) -> [CAN2_USS_Sta_RLL]
  USSStaRLR/1(CAN2_USS_Sta_RLR) -> [CAN2_USS_Sta_RLR]
  USSStaRML/1(CAN2_USS_Sta_RML) -> [CAN2_USS_Sta_RML]
  USSStaRMR/1(CAN2_USS_Sta_RMR) -> [CAN2_USS_Sta_RMR]
  VMCVCUCCCrlSta/1(CAN2_VMC_VCU_CC_Crl_Sta) -> [CAN2_VMC_VCU_CC_Crl_Sta]
  VMCVCUMSACrlSta/1(CAN2_VMC_VCU_MSA_Crl_Sta) -> [CAN2_VMC_VCU_MSA_Crl_Sta]
  bus_selector/1 -> APSExitCondition/1(APSExitCondition)  "<VOUTP_APSExitCondition_enum>"
  [BOUTP_outputs] -> bus_selector/1
  bus_selector1/1 -> APSRQDisplay/1(APSRQDisplay)  "<VOUTP_APSRQDisplay_enum>"
  [BOUTP_outputs] -> bus_selector1/1
  bus_selector2/1 -> APSSWVer/1(APSSWVer)  "<VOUTP_APSSWVer_enum>"
  [BOUTP_outputs] -> bus_selector2/1
  bus_selector3/1 -> APSStaSystem/1(APSStaSystem)  "<VOUTP_APSStaSys_enum>"
  [BOUTP_outputs] -> bus_selector3/1
  bus_selector4/1 -> CAASSta/1(CAASSta)  "<VOUTP_CAASSta_enum>"
  [BOUTP_outputs] -> bus_selector4/1
  bus_selector5/1 -> DISCDISCTargetSpd/1(DISCDISCTargetSpd)  "<VOUTP_DISCTargetSpd_kph>"
  [BOUTP_outputs] -> bus_selector5/1
  bus_selector6/1 -> FDCVCURegenLimIndSta/1(FDCVCURegenLimIndSta)  "<VOUTP_RegenLimIndSta_flg>"
  [BOUTP_outputs] -> bus_selector6/1
  bus_selector7/1 -> FDCVCURegenModeSta/1(FDCVCURegenModeSta)  "<VOUTP_FDCVCURegenMode_enum>"
  [BOUTP_outputs] -> bus_selector7/1
  bus_selector8/1 -> FDCVCUSmartEcoSpdLimSta/1(FDCVCUSmartEcoSpdLimSta)  "<VOUTP_SetSpdLimWarn_flg>"
  [BOUTP_outputs] -> bus_selector8/1
  Ground/1 -> FDCVCUSmartEcoSta/1(FDCVCUSmartEcoSta)
  Ground1/1 -> FDCVMCSetSpdDispSta/1(FDCVMCSetSpdDispSta)
  bus_selector9/1 -> FDCVMCSetSpdSta/1(FDCVMCSetSpdSta)  "<VOUTP_SetSpd_kph>"
  [BOUTP_outputs] -> bus_selector9/1
  bus_selector10/1 -> FDCVMCSpdCtrlModeSta/1(FDCVMCSpdCtrlModeSta)  "<VOUTP_SpdCtrlMode_enum>"
  [BOUTP_outputs] -> bus_selector10/1
  bus_selector11/1 -> FDCVMCSpdCtrlSta/1(FDCVMCSpdCtrlSta)  "<VOUTP_SpdCtrlSta_flg>"
  [BOUTP_outputs] -> bus_selector11/1
  bus_selector12/1 -> PASAFCL/1(PASAFCL)  "<VOUTP_PASAFCL_enum>"
  [BOUTP_outputs] -> bus_selector12/1
  bus_selector13/1 -> PASAFCR/1(PASAFCR)  "<VOUTP_PASAFCR_enum>"
  [BOUTP_outputs] -> bus_selector13/1
  bus_selector14/1 -> PASAFML/1(PASAFML)  "<VOUTP_PASAFML_enum>"
  [BOUTP_outputs] -> bus_selector14/1
  bus_selector15/1 -> PASAFMR/1(PASAFMR)  "<VOUTP_PASAFMR_enum>"
  [BOUTP_outputs] -> bus_selector15/1
  bus_selector16/1 -> PASARCL/1(PASARCL)  "<VOUTP_PASARCL_enum>"
  [BOUTP_outputs] -> bus_selector16/1
  bus_selector17/1 -> PASARCR/1(PASARCR)  "<VOUTP_PASARCR_enum>"
  [BOUTP_outputs] -> bus_selector17/1
  bus_selector18/1 -> PASARML/1(PASARML)  "<VOUTP_PASARML_enum>"
  [BOUTP_outputs] -> bus_selector18/1
  bus_selector19/1 -> PASARMR/1(PASARMR)  "<VOUTP_PASARMR_enum>"
  [BOUTP_outputs] -> bus_selector19/1
  bus_selector20/1 -> PASChime/1(PASChime)  "<VOUTP_Chime_enum>"
  [BOUTP_outputs] -> bus_selector20/1
  bus_selector21/1 -> PASDFCL/1(PASDFCL)  "<VOUTP_PASDFCL_cm>"
  [BOUTP_outputs] -> bus_selector21/1
  bus_selector22/1 -> PASDFCR/1(PASDFCR)  "<VOUTP_PASDFCR_cm>"
  [BOUTP_outputs] -> bus_selector22/1
  bus_selector23/1 -> PASDFML/1(PASDFML)  "<VOUTP_PASDFML_cm>"
  [BOUTP_outputs] -> bus_selector23/1
  bus_selector24/1 -> PASDFMR/1(PASDFMR)  "<VOUTP_PASDFMR_cm>"
  [BOUTP_outputs] -> bus_selector24/1
  bus_selector25/1 -> PASDRCL/1(PASDRCL)  "<VOUTP_PASDRCL_cm>"
  [BOUTP_outputs] -> bus_selector25/1
  bus_selector26/1 -> PASDRCR/1(PASDRCR)  "<VOUTP_PASDRCR_cm>"
  [BOUTP_outputs] -> bus_selector26/1
  bus_selector27/1 -> PASDRML/1(PASDRML)  "<VOUTP_PASDRML_cm>"
  [BOUTP_outputs] -> bus_selector27/1
  bus_selector28/1 -> PASDRMR/1(PASDRMR)  "<VOUTP_PASDRMR_cm>"
  [BOUTP_outputs] -> bus_selector28/1
  bus_selector29/1 -> PASSNSRLayout/1(PASSNSRLayout)  "<VOUTP_SNSRLayout_enum>"
  [BOUTP_outputs] -> bus_selector29/1
  bus_selector30/1 -> USSStaFCL/1(USSStaFCL)  "<VOUTP_USSStaFCL_flg>"
  [BOUTP_outputs] -> bus_selector30/1
  bus_selector31/1 -> USSStaFCR/1(USSStaFCR)  "<VOUTP_USSStaFCR_flg>"
  [BOUTP_outputs] -> bus_selector31/1
  bus_selector32/1 -> USSStaFLL/1(USSStaFLL)  "<VOUTP_USSStaFLL_flg>"
  [BOUTP_outputs] -> bus_selector32/1
  bus_selector33/1 -> USSStaFLR/1(USSStaFLR)  "<VOUTP_USSStaFLR_flg>"
  [BOUTP_outputs] -> bus_selector33/1
  bus_selector34/1 -> USSStaFML/1(USSStaFML)  "<VOUTP_USSStaFML_flg>"
  [BOUTP_outputs] -> bus_selector34/1
  bus_selector35/1 -> USSStaFMR/1(USSStaFMR)  "<VOUTP_USSStaFMR_flg>"
  [BOUTP_outputs] -> bus_selector35/1
  bus_selector36/1 -> USSStaRCL/1(USSStaRCL)  "<VOUTP_USSStaRCL_flg>"
  [BOUTP_outputs] -> bus_selector36/1
  bus_selector37/1 -> USSStaRCR/1(USSStaRCR)  "<VOUTP_USSStaRCR_flg>"
  [BOUTP_outputs] -> bus_selector37/1
  bus_selector38/1 -> USSStaRLL/1(USSStaRLL)  "<VOUTP_USSStaRLL_flg>"
  [BOUTP_outputs] -> bus_selector38/1
  bus_selector39/1 -> USSStaRLR/1(USSStaRLR)  "<VOUTP_USSStaRLR_flg>"
  [BOUTP_outputs] -> bus_selector39/1
  bus_selector40/1 -> USSStaRML/1(USSStaRML)  "<VOUTP_USSStaRML_flg>"
  [BOUTP_outputs] -> bus_selector40/1
  bus_selector41/1 -> USSStaRMR/1(USSStaRMR)  "<VOUTP_USSStaRMR_flg>"
  [BOUTP_outputs] -> bus_selector41/1
  bus_selector42/1 -> VMCVCUCCCrlSta/1(VMCVCUCCCrlSta)  "<VOUTP_CCCtrlSta_enum>"
  [BOUTP_outputs] -> bus_selector42/1
  bus_selector43/1 -> VMCVCUMSACrlSta/1(VMCVCUMSACrlSta)  "<VOUTP_MSACtrlSta_enum>"
  [BOUTP_outputs] -> bus_selector43/1
